simulink model "sensorlessBLDC_2023"  (R2023b)
settings: Solver=VariableStepAuto  StartTime=0.0  StopTime=15  RelTol=1e-3
values from neighbouring files (symbols this model uses):
  Ke = 67.5e-3    (= 0.0675)    [Attitude_OuterLoop.m]    (also in BLDC_measures.m; SystemVariables.m)
  L = 5.2e-3    (= 0.0052)    [Attitude_OuterLoop.m]    (also in BLDC_measures.m; SystemVariables.m)
  R = 5.6    [Attitude_OuterLoop.m]    (also in BLDC_measures.m; SystemVariables.m)
undefined symbols (not defined in the file or in its folder): DiscIntNeverNeededParam, K1, K2, P, Ts
libraries: spsMosfetLib x6, spsCurrentMeasurementLib x3, spsVoltageMeasurementLib x3, spsDCVoltageSourceLib x1, spsPermanentMagnetSynchronousMachineLib x1, simulink x1, hdlsllib x1, slpidlib x1, spspowerguiLib x1
settings Model: Creator=jc02857  LastModifiedBy=jc02857
settings RTWCC: GPUComputeCapability=5.0

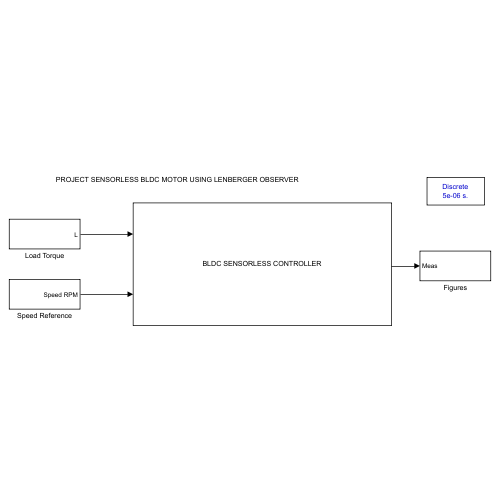
[thumbnail: Simulink's stored preview of the top-level diagram]
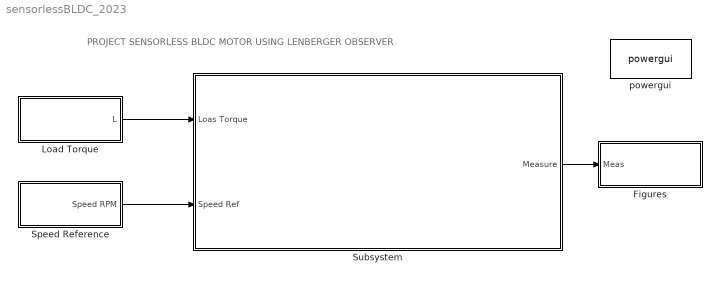
== system sensorlessBLDC_2023 ==
  note: PROJECT SENSORLESS BLDC MOTOR USING LENBERGER OBSERVER
  Figures : Subsystem
  Load Torque : Subsystem
  Speed Reference : Subsystem
  Subsystem : Subsystem
      mask Display: disp('BLDC SENSORLESS CONTROLLER')
  powergui : spspowerguiLib/powergui  Priority=1  SimulationMode=Discrete  SampleTime=5e-6  frequency=60  Iterations=50  frequencyindice=0  Pbase=100e6  ErrMax=1e-4  UnitsV=kV  UnitsW=MW  buscounter=0  FunctionMessages=off  echomessages=off  EnableUseOfTLC=off  CurrentSourceSwitches=off  DisableSnubberDevices=off  DisableRonSwitches=off  DisableVfSwitches=off  DisplayEquations=off  AutomaticDiscreteSolvers=off  SolverType=Tustin/Backward Euler (TBE)  Interpol=off  ExternalGateDelay=off  methode=off  Ts=100  x0status=blocks  SPID=on  SwTol=0  HookPort=off  NonlinearTolerance=1e-4  nMaxIteration=100  ContinueOnMaxIteration=off  RestoreLinks=warning  ResistiveCurrentMeasurement=off  Frange=[0:2:500]  Ylog=off  Xlog=on  ShowGrid=off  save=off  variable=ZData  structure=0  ZoomFFT=off  StartTime=0.0  cycles=1  DisplayStyle=1  fundamental=60  FreqAxis=off  MaxFrequency=1000  frequencyindicesteady=1  RmsSteady=1  display=off
  wires:
  Speed Reference/1(Speed RPM) -> Subsystem/2(Speed Ref)
  Subsystem/1(Measure) -> Figures/1(Meas)
  Load Torque/1(L) -> Subsystem/1(Loas Torque)

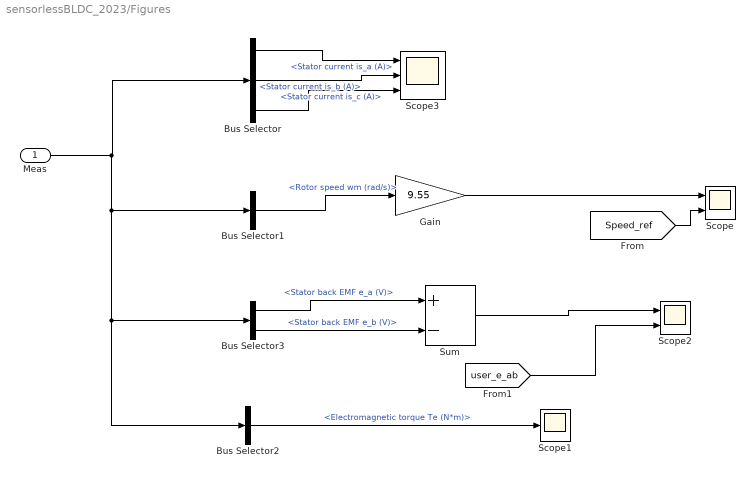
== system sensorlessBLDC_2023/Figures ==
  Meas : Inport
  Bus Selector : BusSelector  OutputSignals=Stator current is_a (A),Stator current is_b (A),Stator current is_c (A)
  Bus Selector1 : BusSelector  OutputSignals=Rotor speed wm (rad/s)
  Bus Selector2 : BusSelector  OutputSignals=Electromagnetic torque Te (N*m)
  Bus Selector3 : BusSelector  OutputSignals=Stator back EMF e_a (V),Stator back EMF e_b (V)
  Gain : Gain  Gain=9.55
  Scope : Scope  NumInputPorts=2
  Scope1 : Scope
  Scope2 : Scope  NumInputPorts=2
  Scope3 : Scope  NumInputPorts=3
  Sum : Sum  Inputs=+-
  wires:
  Meas/1 -> Bus Selector3/1, Bus Selector2/1, Bus Selector1/1, Bus Selector/1
  Bus Selector1/1 -> Gain/1  "<Rotor speed wm (rad/s)>"
  Gain/1 -> Scope/1
  [Speed_ref] -> Scope/2
  Bus Selector2/1 -> Scope1/1  "<Electromagnetic torque Te (N*m)>"
  Bus Selector3/1 -> Sum/1  "<Stator back EMF e_a (V)>"
  Bus Selector3/2 -> Sum/2  "<Stator back EMF e_b (V)>"
  Sum/1 -> Scope2/1
  [user_e_ab] -> Scope2/2
  Bus Selector/1 -> Scope3/1  "<Stator current is_a (A)>"
  Bus Selector/2 -> Scope3/2  "<Stator current is_b (A)>"
  Bus Selector/3 -> Scope3/3  "<Stator current is_c (A)>"

== system sensorlessBLDC_2023/Load Torque ==
  Constant : Constant  Value=0
  Load Torque : Step  SampleTime=0
  Manual Switch : ManualSwitch
  L : Outport
  wires:
  Constant/1 -> Manual Switch/1
  Load Torque/1 -> Manual Switch/2
  Manual Switch/1 -> [Load], L/1

== system sensorlessBLDC_2023/Speed Reference ==
  1000rpm : Constant  Value=2000
  Manual Switch : ManualSwitch
  RPM : Constant  Value=-50
  Speed RPM : Outport
  tag scope: Speed_ref=global
  wires:
  1000rpm/1 -> Manual Switch/2
  RPM/1 -> Manual Switch/1
  Manual Switch/1 -> [Speed_ref], Speed RPM/1

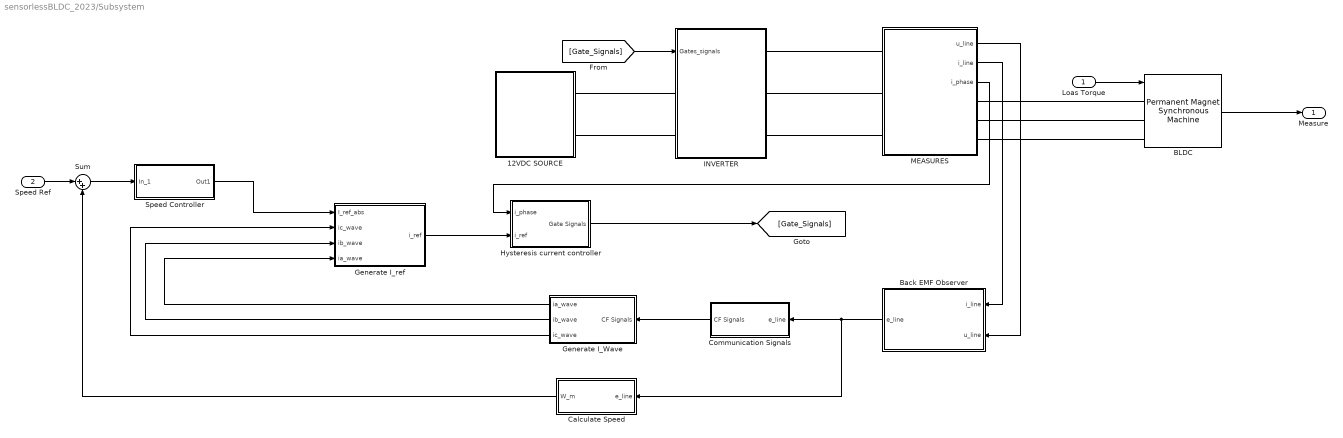
== system sensorlessBLDC_2023/Subsystem ==
  Loas Torque : Inport
  Speed Ref : Inport  Port=2
  12VDC SOURCE : Subsystem
  BLDC : spsPermanentMagnetSynchronousMachineLib/Permanent Magnet Synchronous Machine  NbPhases=3  FluxDistribution=Trapezoidal  RotorType=Round  MechanicalLoad=Torque Tm  PresetModel=No  ShowDetailedParameters=on  MeasurementBus=off  Resistance=5.6  Inductance=5.2e-3  dqInductances=[8.5e-3,8.5e-3]  La=0.000395  MachineConstant=Torque Constant (N.m / A_peak)  Flux=0.0030682  VoltageCst=7.0686  TorqueCst=67.5e-3  Flat=120  Mechanical=[0.00254 10e-6 11 0]  PolePairs=4  InitialConditions=[0,0, 0,0]  InitialConditions5ph=[0 0 0 0 0 0]  RefAngle=Aligned with phase A axis (original Park)  IterativeDiscreteModel=Trapezoidal non iterative  TsBlock=-1  TsPowergui=0
  Back EMF Observer : Subsystem
  Calculate Speed : Subsystem
  Communication Signals : Subsystem
  Generate I_Wave : Subsystem
  Generate I_ref : Subsystem
  Hysteresis current controller : Subsystem  mask{h=0}
      mask prompts: h "Hysteresis band"
  INVERTER : Subsystem
  MEASURES : Subsystem
  Speed Controller : Subsystem  mask{I=0.89, P=13, sat=[-15, 15]}
      mask prompts: I "Integral"; P "Proportional"; sat "min max"
      mask Display: disp('PI Controller')
  Sum : Sum  Inputs=|++
  Measure : Outport
  wires:
  BLDC/1 -> Measure/1
  MEASURES/1(u_line) -> Back EMF Observer/2(u_line)
  Loas Torque/1 -> BLDC/1
  Speed Ref/1 -> Sum/1
  Communication Signals/1("CF Signals  ") -> Generate I_Wave/1(CF Signals)
  Speed Controller/1(Out1) -> Generate I_ref/1(I_ref_abs)
  [Gate_Signals] -> INVERTER/1(Gates_signals)
  Sum/1 -> Speed Controller/1(In_1)
  MEASURES/2(i_line) -> Back EMF Observer/1(i_line)
  Generate I_ref/1(i_ref) -> Hysteresis current controller/2(i_ref)
  Back EMF Observer/1(e_line) -> Calculate Speed/1(e_line), Communication Signals/1(e_line)
  Generate I_Wave/1(ia_wave) -> Generate I_ref/4(ia_wave)
  Generate I_Wave/3(ic_wave) -> Generate I_ref/2(ic_wave)
  Generate I_Wave/2(ib_wave) -> Generate I_ref/3(ib_wave)
  MEASURES/3(i_phase) -> Hysteresis current controller/1(i_phase)
  Calculate Speed/1(W_m) -> Sum/2
  Hysteresis current controller/1(Gate Signals) -> [Gate_Signals]
  connections:
  BLDC/LConn2 -- MEASURES/RConn2
  INVERTER/RConn3 -- MEASURES/LConn3
  MEASURES/RConn1 -- BLDC/LConn1
  BLDC/LConn3 -- MEASURES/RConn3
  12VDC SOURCE/RConn1 -- INVERTER/LConn1
  INVERTER/RConn1 -- MEASURES/LConn1
  MEASURES/LConn2 -- INVERTER/RConn2
  12VDC SOURCE/RConn2 -- INVERTER/LConn2

== system sensorlessBLDC_2023/Subsystem/12VDC SOURCE ==
  DC Voltage Source : spsDCVoltageSourceLib/DC Voltage Source  Amplitude=11.1  Measurements=None
  Positive : PMIOPort  Side=Right
  Negative : PMIOPort  Port=2  Side=Right
  connections:
  Positive/RConn1 -- DC Voltage Source/RConn1
  Negative/RConn1 -- DC Voltage Source/LConn1

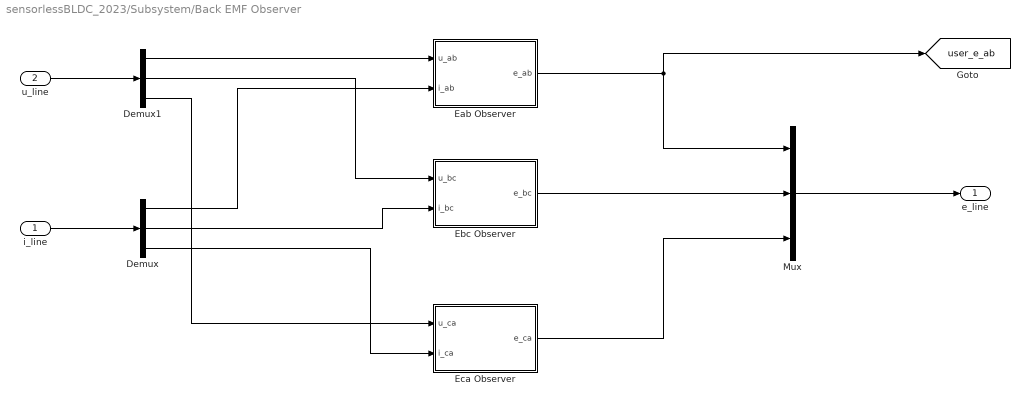
== system sensorlessBLDC_2023/Subsystem/Back EMF Observer ==
  i_line : Inport
  u_line : Inport  Port=2
  Demux : Demux  Outputs=3
  Demux1 : Demux  Outputs=3
  Eab Observer : Subsystem
  Ebc Observer : Subsystem
  Eca Observer : Subsystem
  Mux : Mux  Inputs=3
  e_line : Outport
  tag scope: user_e_ab=global
  wires:
  i_line/1 -> Demux/1
  u_line/1 -> Demux1/1
  Demux1/1 -> Eab Observer/1(u_ab)
  Demux/1 -> Eab Observer/2(i_ab)
  Demux1/2 -> Ebc Observer/1(u_bc)
  Demux1/3 -> Eca Observer/1(u_ca)
  Demux/2 -> Ebc Observer/2(i_bc)
  Demux/3 -> Eca Observer/2(i_ca)
  Ebc Observer/1(e_bc) -> Mux/2
  Eab Observer/1(e_ab) -> Mux/1, [user_e_ab]
  Eca Observer/1(e_ca) -> Mux/3
  Mux/1 -> e_line/1

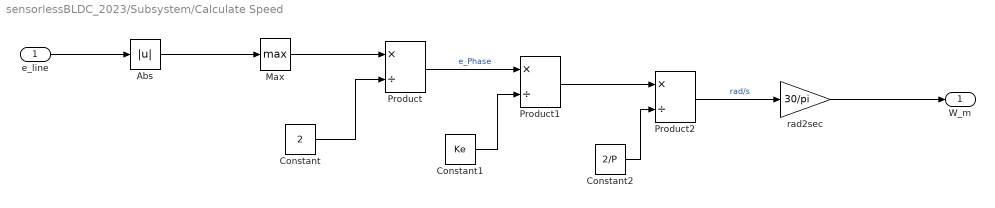
== system sensorlessBLDC_2023/Subsystem/Calculate Speed ==
  e_line : Inport
  Abs : Abs  SaturateOnIntegerOverflow=off
  Constant : Constant  Value=2
  Constant1 : Constant  Value=Ke
  Constant2 : Constant  Value=2/P
  Max : MinMax  Function=max
  Product : Product  Inputs=*/
  Product1 : Product  Inputs=*/
  Product2 : Product  Inputs=*/
  rad2sec : Gain  Gain=30/pi
  W_m : Outport
  wires:
  e_line/1 -> Abs/1
  Abs/1 -> Max/1
  Max/1 -> Product/1
  Constant/1 -> Product/2
  Product/1 -> Product1/1  "e_Phase"
  Constant1/1 -> Product1/2
  Product1/1 -> Product2/1
  Constant2/1 -> Product2/2
  Product2/1 -> rad2sec/1  "rad/s"
  rad2sec/1 -> W_m/1

== system sensorlessBLDC_2023/Subsystem/Communication Signals ==
  e_line : Inport
  CF Signals : Subsystem
  Demux : Demux  Outputs=3
  Detect Rise Positive : simulink/Logic and Bit Operations/Detect Rise Positive  vinit=0  OutDataTypeStr=boolean
  Product : Product  Inputs=*/
  Product1 : Product  Inputs=*/
  Product2 : Product  Inputs=*/
  Sum : Sum  Inputs=+++
  "CF Signals  " : Outport
  wires:
  e_line/1 -> Demux/1
  Demux/1 -> Product2/2, Product1/1  "eab"
  Demux/2 -> Product1/2, Product/1  "ebc"
  Demux/3 -> Product2/1, Product/2  "eca"
  Product1/1 -> Sum/2
  Product/1 -> Sum/1
  Product2/1 -> Sum/3
  Sum/1 -> Detect Rise Positive/1
  Detect Rise Positive/1 -> CF Signals/Trigger
  CF Signals/1(Out1) -> "CF Signals  "/1

== system sensorlessBLDC_2023/Subsystem/Generate I_Wave ==
  CF Signals : Inport
  COUNTER SIGNALS : Subsystem
  Constant : Constant  Value=6
  Generate wave : Subsystem
  Rem : Math  Operator=rem
  ia_wave : Outport
  ib_wave : Outport  Port=2
  ic_wave : Outport  Port=3
  wires:
  Constant/1 -> Rem/2
  COUNTER SIGNALS/1(Counter) -> Rem/1
  Rem/1 -> Generate wave/1(Mode)
  CF Signals/1 -> COUNTER SIGNALS/Trigger
  Generate wave/1(ia_wave) -> ia_wave/1
  Generate wave/2(ib_wave) -> ib_wave/1
  Generate wave/3(ic_wave) -> ic_wave/1

== system sensorlessBLDC_2023/Subsystem/Generate I_ref ==
  I_ref_abs : Inport
  ic_wave : Inport  Port=2
  ib_wave : Inport  Port=3
  ia_wave : Inport  Port=4
  Mux : Mux  Inputs=3
  Product : Product
  Product1 : Product
  Product2 : Product
  i_ref : Outport
  wires:
  ia_wave/1 -> Product/1
  I_ref_abs/1 -> Product2/2, Product1/2, Product/2
  ib_wave/1 -> Product1/1
  ic_wave/1 -> Product2/1
  Product/1 -> Mux/1
  Product1/1 -> Mux/2
  Product2/1 -> Mux/3
  Mux/1 -> i_ref/1

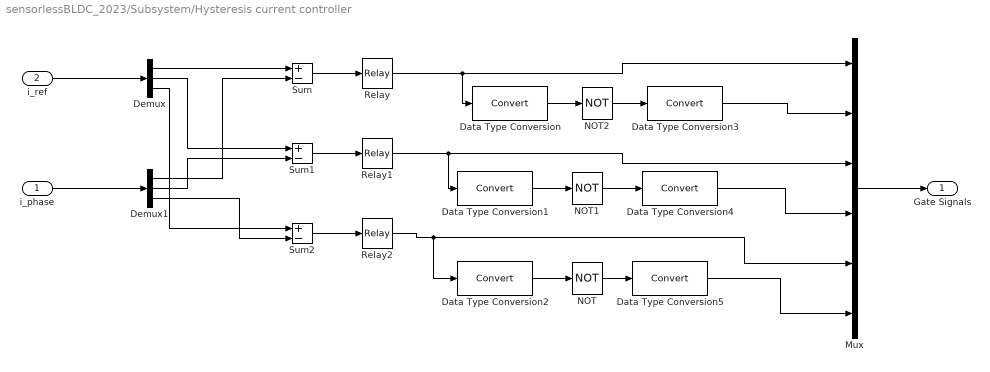
== system sensorlessBLDC_2023/Subsystem/Hysteresis current controller ==
  i_phase : Inport
  i_ref : Inport  Port=2
  Data Type Conversion{,1..5} (6 alike) : DataTypeConversion  SaturateOnIntegerOverflow=off  RndMeth=Floor
  Demux : Demux  Outputs=3
  Demux1 : Demux  Outputs=3
  Mux : Mux  Inputs=6
  NOT : Logic  Operator=NOT  IconShape=distinctive  AllPortsSameDT=off  OutDataTypeStr=boolean
  NOT1 : Logic  Operator=NOT  IconShape=distinctive  AllPortsSameDT=off  OutDataTypeStr=boolean
  NOT2 : Logic  Operator=NOT  IconShape=distinctive  AllPortsSameDT=off  OutDataTypeStr=boolean
  Relay : Relay
  Relay1 : Relay
  Relay2 : Relay
  Sum : Sum  Inputs=+-
  Sum1 : Sum  Inputs=+-
  Sum2 : Sum  Inputs=+-
  Gate Signals : Outport
  wires:
  i_ref/1 -> Demux/1
  i_phase/1 -> Demux1/1
  Demux/1 -> Sum/1
  Demux1/1 -> Sum/2
  Demux/2 -> Sum1/1
  Demux1/2 -> Sum1/2
  Demux/3 -> Sum2/1
  Demux1/3 -> Sum2/2
  Sum2/1 -> Relay2/1
  Sum1/1 -> Relay1/1
  Sum/1 -> Relay/1
  Data Type Conversion2/1 -> NOT/1
  Data Type Conversion1/1 -> NOT1/1
  Data Type Conversion/1 -> NOT2/1
  NOT2/1 -> Data Type Conversion3/1
  NOT1/1 -> Data Type Conversion4/1
  NOT/1 -> Data Type Conversion5/1
  Mux/1 -> Gate Signals/1
  Relay/1 -> Data Type Conversion/1, Mux/1
  Data Type Conversion3/1 -> Mux/2
  Data Type Conversion4/1 -> Mux/4
  Data Type Conversion5/1 -> Mux/6
  Relay2/1 -> Mux/5, Data Type Conversion2/1
  Relay1/1 -> Data Type Conversion1/1, Mux/3

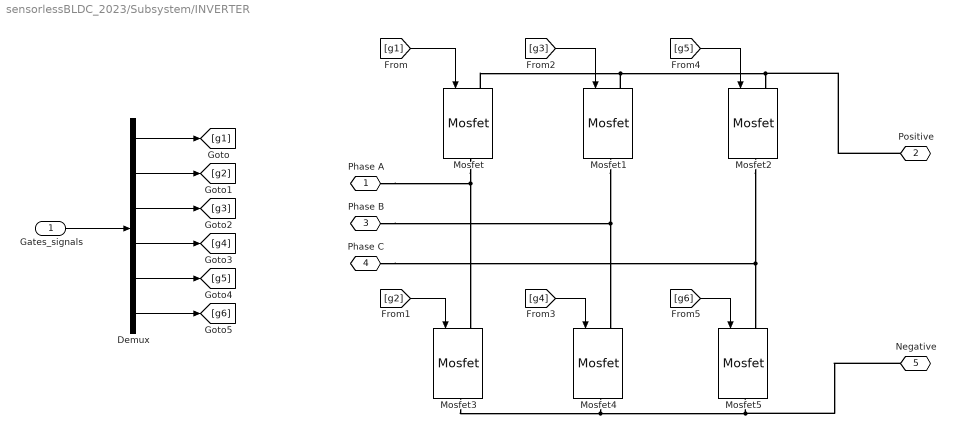
== system sensorlessBLDC_2023/Subsystem/INVERTER ==
  Gates_signals : Inport
  Demux : Demux  Outputs=6
  Mosfet{,1..5} (6 alike) : spsMosfetLib/Mosfet  Ron=0.006/95  Lon=0  Rd=0.01  Vfd=0  IC=0  Rs=10e03  Cs=inf  Measurements=off
  Phase A : PMIOPort  Side=Right
  Positive : PMIOPort  Port=2  Side=Left
  Phase B : PMIOPort  Port=3  Side=Right
  Phase C : PMIOPort  Port=4  Side=Right
  Negative : PMIOPort  Port=5  Side=Left
  wires:
  [g1] -> Mosfet/1
  [g2] -> Mosfet3/1
  [g3] -> Mosfet1/1
  [g4] -> Mosfet4/1
  [g6] -> Mosfet5/1
  [g5] -> Mosfet2/1
  Gates_signals/1 -> Demux/1
  Demux/1 -> [g1]
  Demux/6 -> [g6]
  Demux/5 -> [g5]
  Demux/4 -> [g4]
  Demux/3 -> [g3]
  Demux/2 -> [g2]
  connections:
  Mosfet2/RConn1 -- Phase C/RConn1 -- Mosfet5/LConn1
  Mosfet1/RConn1 -- Mosfet4/LConn1 -- Phase B/RConn1
  Mosfet/RConn1 -- Mosfet3/LConn1 -- Phase A/RConn1
  Mosfet/LConn1 -- Mosfet1/LConn1 -- Positive/RConn1 -- Mosfet2/LConn1
  Mosfet3/RConn1 -- Mosfet4/RConn1 -- Negative/RConn1 -- Mosfet5/RConn1

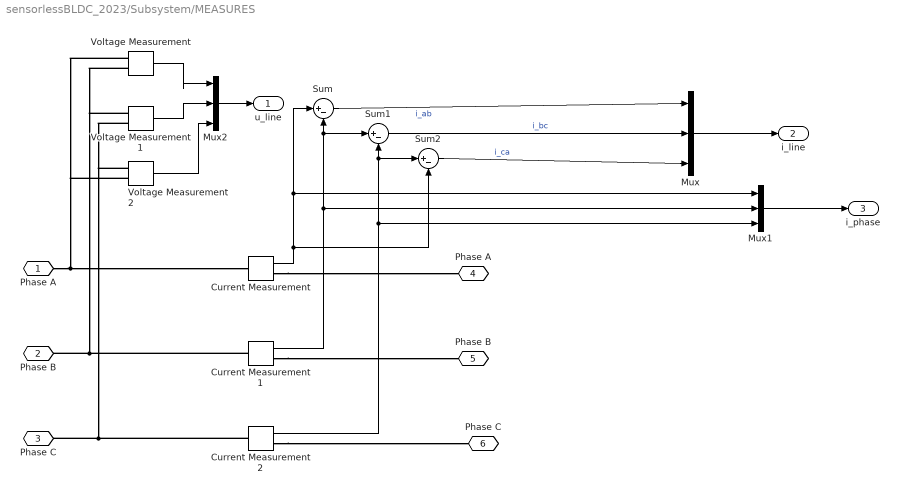
== system sensorlessBLDC_2023/Subsystem/MEASURES ==
  Current Measurement : spsCurrentMeasurementLib/Current Measurement  PhasorSimulation=off  OutputType=Complex  PSBequivalent=0
  Current Measurement1 : spsCurrentMeasurementLib/Current Measurement  PhasorSimulation=off  OutputType=Complex  PSBequivalent=0
  Current Measurement2 : spsCurrentMeasurementLib/Current Measurement  PhasorSimulation=off  OutputType=Complex  PSBequivalent=0
  Mux : Mux  Inputs=3
  Mux1 : Mux  Inputs=3
  Mux2 : Mux  Inputs=3
  Sum : Sum  Inputs=|+-
  Sum1 : Sum  Inputs=|+-
  Sum2 : Sum  Inputs=|+-
  Voltage Measurement : spsVoltageMeasurementLib/Voltage Measurement  PhasorSimulation=off  OutputType=Complex  PSBequivalent=0
  Voltage Measurement1 : spsVoltageMeasurementLib/Voltage Measurement  PhasorSimulation=off  OutputType=Complex  PSBequivalent=0
  Voltage Measurement2 : spsVoltageMeasurementLib/Voltage Measurement  PhasorSimulation=off  OutputType=Complex  PSBequivalent=0
  "Phase A  " : PMIOPort  Side=Left
  Phase B : PMIOPort  Port=2  Side=Left
  Phase C : PMIOPort  Port=3  Side=Left
  Phase A : PMIOPort  Port=4  Side=Right
  "Phase B  " : PMIOPort  Port=5  Side=Right
  "Phase C  " : PMIOPort  Port=6  Side=Right
  u_line : Outport
  i_line : Outport  Port=2
  i_phase : Outport  Port=3
  wires:
  Current Measurement/1 -> Sum2/2, Sum/1, Mux1/1
  Current Measurement1/1 -> Mux1/2, Sum1/1, Sum/2
  Sum/1 -> Mux/1  "i_ab"
  Current Measurement2/1 -> Sum2/1, Sum1/2, Mux1/3
  Sum1/1 -> Mux/2  "i_bc"
  Sum2/1 -> Mux/3  "i_ca"
  Mux/1 -> i_line/1
  Mux1/1 -> i_phase/1
  Voltage Measurement/1 -> Mux2/1
  Voltage Measurement1/1 -> Mux2/2
  Voltage Measurement2/1 -> Mux2/3
  Mux2/1 -> u_line/1
  connections:
  Current Measurement/RConn1 -- Phase A/RConn1
  "Phase A  "/RConn1 -- Voltage Measurement2/LConn2 -- Voltage Measurement/LConn1 -- Current Measurement/LConn1
  Current Measurement1/LConn1 -- Voltage Measurement/LConn2 -- Voltage Measurement1/LConn1 -- Phase B/RConn1
  Current Measurement2/LConn1 -- Voltage Measurement2/LConn1 -- Voltage Measurement1/LConn2 -- Phase C/RConn1
  Current Measurement1/RConn1 -- "Phase B  "/RConn1
  Current Measurement2/RConn1 -- "Phase C  "/RConn1

== system sensorlessBLDC_2023/Subsystem/Speed Controller ==
  note: Tuner836f4fdf618b
  note: Tunerd399ab9cd8bd
  note: Tuner04e83206f1f0
  note: Tuner4f26d6e2d051
  In_1 : Inport
  Gain : Gain  Gain=P
  PID Controller : slpidlib/PID Controller  Controller=PI  Form=Parallel  TimeDomain=Continuous-time  UseExternalTs=off  SampleTime=-1  IntegratorMethod=Forward Euler  FilterMethod=Forward Euler  ControllerParametersSource=internal  P=0  I=14.3446  UseKiTs=off  D=0.0024799  N=6000  UseFilter=on  TunerSelectOption=Frequency Response Based  InitialConditionSource=internal  InitialConditionForIntegrator=0  InitialConditionForFilter=0  DifferentiatorICPrevScaledInput=0  ExternalReset=none  TrackingMode=off  Kt=1  LimitOutput=off  SatLimitsSource=internal  UpperSaturationLimit=inf  LowerSaturationLimit=-inf  LinearizeAsGain=on  AntiWindupMode=none  Kb=1  LimitIntegrator=off  UpperIntegratorSaturationLimit=inf  LowerIntegratorSaturationLimit=-inf  POutMin=[]  POutMax=[]  IOutMin=[]  IOutMax=[]  DOutMin=[]  DOutMax=[]  NOutMin=[]  NOutMax=[]  SumOutMin=[]  SumOutMax=[]  SaturationOutMin=[]  SaturationOutMax=[]  PParamMin=[]  PParamMax=[]  IParamMin=[]  IParamMax=[]  DParamMin=[]  DParamMax=[]  NParamMin=[]  NParamMax=[]  KbParamMin=[]  KbParamMax=[]  KtParamMin=[]  KtParamMax=[]  KbOutMin=[]  KbOutMax=[]  KtOutMin=[]  KtOutMax=[]  IntegratorOutMin=[]  IntegratorOutMax=[]  FilterOutMin=[]  FilterOutMax=[]  SumI1OutMin=[]  SumI1OutMax=[]  SumI2OutMin=[]  SumI2OutMax=[]  SumI3OutMin=[]  SumI3OutMax=[]  SumI4OutMin=[]  SumI4OutMax=[]  SumDOutMin=[]  SumDOutMax=[]  DifferentiatorOutMin=[]  DifferentiatorOutMax=[]  FilterDiffOutCoefMin=[]  FilterDiffOutCoefMax=[]  ReciprocalOutMin=[]  ReciprocalOutMax=[]  SumDenOutMin=[]  SumDenOutMax=[]  SumNumOutMin=[]  SumNumOutMax=[]  DivideOutMin=[]  DivideOutMax=[]  UdiffTsProdOutMin=[]  UdiffTsProdOutMax=[]  NTsProdOutMin=[]  NTsProdOutMax=[]  UintegralTsProdOutMin=[]  UintegralTsProdOutMax=[]  UngainTsProdOutMin=[]  UngainTsProdOutMax=[]  ClampingZeroOutDataTypeStr=Inherit: Inherit via back propagation  ClampingZeroOutMin=[]  ClampingZeroOutMax=[]  FilterDenConstantOutDataTypeStr=Inherit: Inherit via back propagation  FilterDenConstantOutMin=[]  FilterDenConstantOutMax=[]  PCopyOutDataTypeStr=Inherit: Inherit via back propagation  PCopyOutMin=[]  PCopyOutMax=[]  NCopyOutDataTypeStr=Inherit: Inherit via back propagation  NCopyOutMin=[]  NCopyOutMax=[]  IntegratorContinuousStateAttributes=''  IntegratorStateMustResolveToSignalObject=off  IntegratorRTWStateStorageClass=Auto  FilterContinuousStateAttributes=''  FilterStateMustResolveToSignalObject=off  FilterRTWStateStorageClass=Auto  ParallelPVariant=InternalParameters  IdealPVariant=Disabled  IVariant=InternalParameters  DVariant=Disabled  IntegratorVariant=Continuous  SatVariant=Disabled  AWVariant=Passthrough  PCopyVariant=Disabled  TRVariant=Disabled  FdbkBlocksVariant=Forward  IdealPFdbkVariant=Disabled  SatFdbkVariant=Disabled  DerivativeFilterVariant=Disabled  NVariant=Disabled  NCopyVariant=Disabled_SignalSpec  FilterICVariant=Disabled  IntegratorICVariant=InternalICs  ExternalResetVariant=Disabled  TRSumVariant=Passthrough  SumFdbkVariant=Disabled  SumVariant=Sum_PI  TsampFilterVariant=InternalTs  TsampNgainVariant=Passthrough  TsampIntegralVariant=Disabled_SignalSpec  ExternalSaturationOutDataTypeStr=Inherit: Same as second input
  Saturation : Saturate  UpperLimit=11  LowerLimit=-11
  Sum : Sum  Inputs=|++
  Transfer Fcn : TransferFcn  Numerator=[I]  Denominator=[1 0]
  Out1 : Outport
  wires:
  Transfer Fcn/1 -> Sum/2
  Saturation/1 -> Out1/1
  Gain/1 -> Sum/1
  PID Controller/1 -> Saturation/1
  In_1/1 -> PID Controller/1

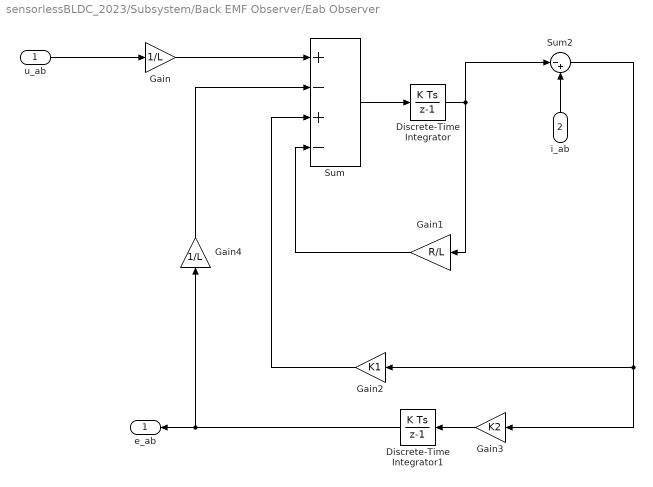
== system sensorlessBLDC_2023/Subsystem/Back EMF Observer/Eab Observer ==
  u_ab : Inport
  i_ab : Inport  Port=2
  Discrete-Time Integrator : DiscreteIntegrator  SampleTime=Ts  ICPrevOutput=DiscIntNeverNeededParam  ICPrevScaledInput=DiscIntNeverNeededParam
  Discrete-Time Integrator1 : DiscreteIntegrator  SampleTime=Ts  ICPrevOutput=DiscIntNeverNeededParam  ICPrevScaledInput=DiscIntNeverNeededParam
  Gain : Gain  Gain=1/L
  Gain1 : Gain  Gain=R/L
  Gain2 : Gain  Gain=K1
  Gain3 : Gain  Gain=K2
  Gain4 : Gain  Gain=1/L
  Sum : Sum  Inputs=+-+-
  Sum2 : Sum  Inputs=|-+
  e_ab : Outport
  wires:
  u_ab/1 -> Gain/1
  Gain/1 -> Sum/1
  Sum/1 -> Discrete-Time Integrator/1
  Discrete-Time Integrator/1 -> Sum2/1, Gain1/1
  Gain1/1 -> Sum/4
  Sum2/1 -> Gain2/1, Gain3/1
  Gain2/1 -> Sum/3
  i_ab/1 -> Sum2/2
  Gain3/1 -> Discrete-Time Integrator1/1
  Discrete-Time Integrator1/1 -> Gain4/1, e_ab/1
  Gain4/1 -> Sum/2

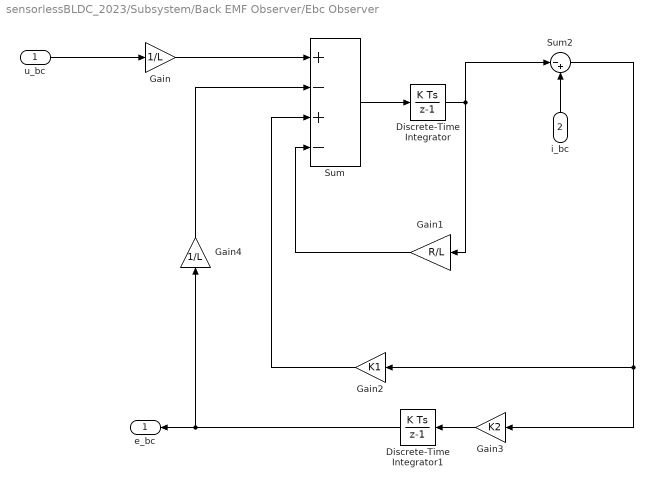
== system sensorlessBLDC_2023/Subsystem/Back EMF Observer/Ebc Observer ==
  u_bc : Inport
  i_bc : Inport  Port=2
  Discrete-Time Integrator : DiscreteIntegrator  SampleTime=Ts  ICPrevOutput=DiscIntNeverNeededParam  ICPrevScaledInput=DiscIntNeverNeededParam
  Discrete-Time Integrator1 : DiscreteIntegrator  SampleTime=Ts  ICPrevOutput=DiscIntNeverNeededParam  ICPrevScaledInput=DiscIntNeverNeededParam
  Gain : Gain  Gain=1/L
  Gain1 : Gain  Gain=R/L
  Gain2 : Gain  Gain=K1
  Gain3 : Gain  Gain=K2
  Gain4 : Gain  Gain=1/L
  Sum : Sum  Inputs=+-+-
  Sum2 : Sum  Inputs=|-+
  e_bc : Outport
  wires:
  u_bc/1 -> Gain/1
  Gain/1 -> Sum/1
  Sum/1 -> Discrete-Time Integrator/1
  Discrete-Time Integrator/1 -> Sum2/1, Gain1/1
  Gain1/1 -> Sum/4
  Sum2/1 -> Gain2/1, Gain3/1
  Gain2/1 -> Sum/3
  i_bc/1 -> Sum2/2
  Gain3/1 -> Discrete-Time Integrator1/1
  Discrete-Time Integrator1/1 -> Gain4/1, e_bc/1
  Gain4/1 -> Sum/2

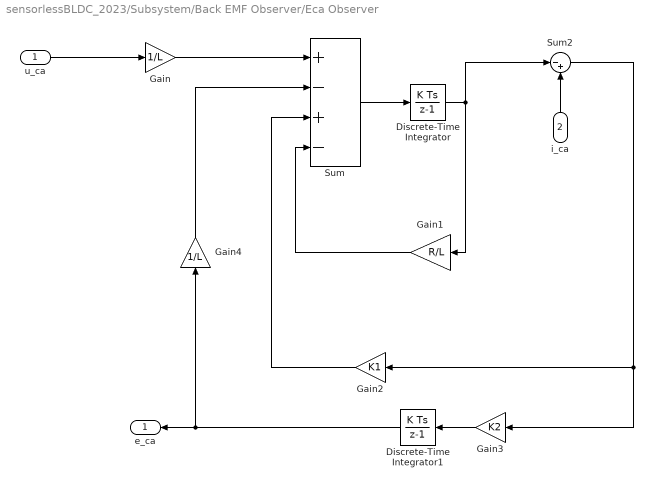
== system sensorlessBLDC_2023/Subsystem/Back EMF Observer/Eca Observer ==
  u_ca : Inport
  i_ca : Inport  Port=2
  Discrete-Time Integrator : DiscreteIntegrator  SampleTime=Ts  ICPrevOutput=DiscIntNeverNeededParam  ICPrevScaledInput=DiscIntNeverNeededParam
  Discrete-Time Integrator1 : DiscreteIntegrator  SampleTime=Ts  ICPrevOutput=DiscIntNeverNeededParam  ICPrevScaledInput=DiscIntNeverNeededParam
  Gain : Gain  Gain=1/L
  Gain1 : Gain  Gain=R/L
  Gain2 : Gain  Gain=K1
  Gain3 : Gain  Gain=K2
  Gain4 : Gain  Gain=1/L
  Sum : Sum  Inputs=+-+-
  Sum2 : Sum  Inputs=|-+
  e_ca : Outport
  wires:
  u_ca/1 -> Gain/1
  Gain/1 -> Sum/1
  Sum/1 -> Discrete-Time Integrator/1
  Discrete-Time Integrator/1 -> Sum2/1, Gain1/1
  Gain1/1 -> Sum/4
  Sum2/1 -> Gain2/1, Gain3/1
  Gain2/1 -> Sum/3
  i_ca/1 -> Sum2/2
  Gain3/1 -> Discrete-Time Integrator1/1
  Discrete-Time Integrator1/1 -> Gain4/1, e_ca/1
  Gain4/1 -> Sum/2

== system sensorlessBLDC_2023/Subsystem/Communication Signals/CF Signals ==
  Trigger : TriggerPort  VariantControl=(inherit)  PortDimensions=1
  Constant : Constant
  Memory : Memory  InheritSampleTime=on
  Sum : Sum  Inputs=|+-
  Out1 : Outport
  wires:
  Constant/1 -> Sum/1
  Memory/1 -> Sum/2
  Sum/1 -> Memory/1, Out1/1

== system sensorlessBLDC_2023/Subsystem/Generate I_Wave/COUNTER SIGNALS ==
  Trigger : TriggerPort  TriggerType=either  VariantControl=(inherit)  PortDimensions=1
  Constant : Constant  Value=0
  Increment Stored Integer : hdlsllib/Math Operations/Increment Stored Integer
  Sum : Sum  Inputs=|++
  Unit Delay : UnitDelay  SampleTime=-1  HasFrameUpgradeWarning=on
  Counter : Outport
  wires:
  Constant/1 -> Sum/1
  Unit Delay/1 -> Sum/2
  Sum/1 -> Increment Stored Integer/1
  Increment Stored Integer/1 -> Unit Delay/1, Counter/1

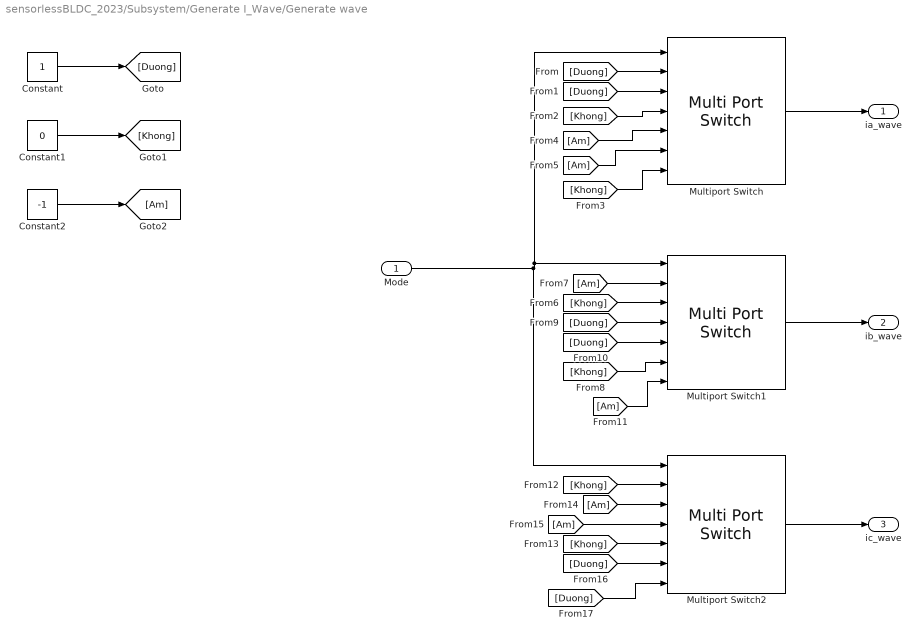
== system sensorlessBLDC_2023/Subsystem/Generate I_Wave/Generate wave ==
  Mode : Inport
  Constant : Constant
  Constant1 : Constant  Value=0
  Constant2 : Constant  Value=-1
  Multiport Switch : MultiPortSwitch  DataPortOrder=Specify indices  DataPortIndices={0,1,2,3,4,5}  SaturateOnIntegerOverflow=off  InputSameDT=off
  Multiport Switch1 : MultiPortSwitch  DataPortOrder=Specify indices  DataPortIndices={0,1,2,3,4,5}  SaturateOnIntegerOverflow=off  InputSameDT=off
  Multiport Switch2 : MultiPortSwitch  DataPortOrder=Specify indices  DataPortIndices={0,1,2,3,4,5}  SaturateOnIntegerOverflow=off  InputSameDT=off
  ia_wave : Outport
  ib_wave : Outport  Port=2
  ic_wave : Outport  Port=3
  wires:
  Constant/1 -> [Duong]
  Constant2/1 -> [Am]
  Constant1/1 -> [Khong]
  Multiport Switch/1 -> ia_wave/1
  Multiport Switch1/1 -> ib_wave/1
  Multiport Switch2/1 -> ic_wave/1
  Mode/1 -> Multiport Switch2/1, Multiport Switch1/1, Multiport Switch/1
  [Duong] -> Multiport Switch/2
  [Duong] -> Multiport Switch/3
  [Khong] -> Multiport Switch/4
  [Khong] -> Multiport Switch/7
  [Am] -> Multiport Switch/5
  [Am] -> Multiport Switch/6
  [Khong] -> Multiport Switch1/6
  [Am] -> Multiport Switch1/2
  [Khong] -> Multiport Switch1/3
  [Duong] -> Multiport Switch1/4
  [Duong] -> Multiport Switch1/5
  [Am] -> Multiport Switch1/7
  [Khong] -> Multiport Switch2/2
  [Khong] -> Multiport Switch2/5
  [Am] -> Multiport Switch2/3
  [Am] -> Multiport Switch2/4
  [Duong] -> Multiport Switch2/6
  [Duong] -> Multiport Switch2/7
